simulink model "Lab1"  (R2021a)
settings: Solver=VariableStepAuto  StartTime=0.0  StopTime=8  RelTol=1e-3
undefined symbols (not defined in the file or in its folder): square
libraries: simulink x4
settings Model: Creator=alsin  LastModifiedBy=yasse

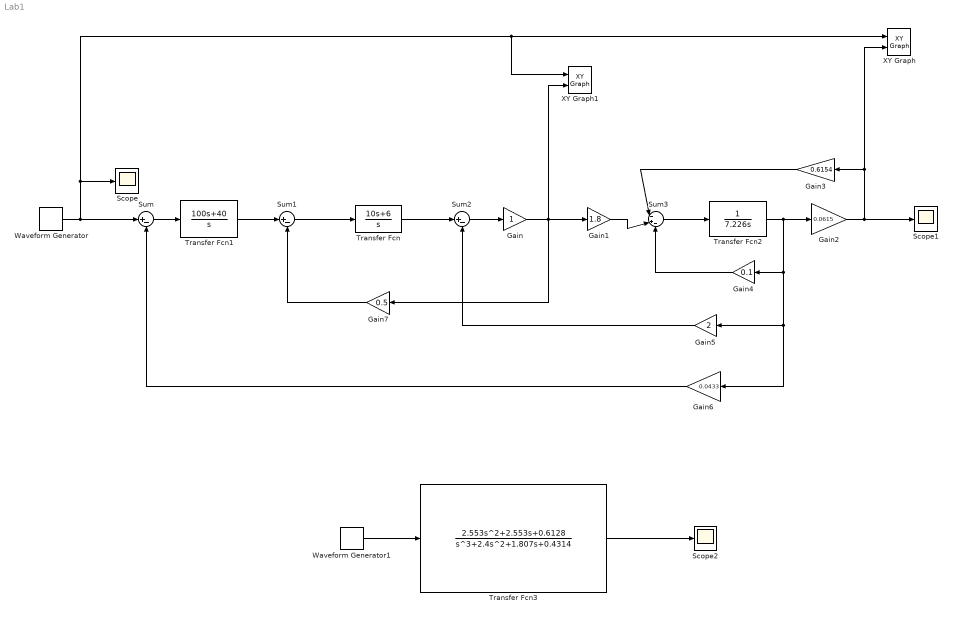
== system Lab1 ==
  Gain : Gain
  Gain1 : Gain  Gain=1.8
  Gain2 : Gain  Gain=0.0615
  Gain3 : Gain  Gain=0.6154
  Gain4 : Gain  Gain=0.1
  Gain5 : Gain  Gain=2
  Gain6 : Gain  Gain=0.0433
  Gain7 : Gain  Gain=0.5
  Scope : Scope
  Scope1 : Scope
  Scope2 : Scope
  Sum : Sum  Inputs=|+-
  Sum1 : Sum  Inputs=|+-
  Sum2 : Sum  Inputs=|+-
  Sum3 : Sum  Inputs=|-+-
  Transfer Fcn : TransferFcn  Numerator=[10 6]  Denominator=[1 0]  ContinuousStateAttributes='KaGtc'
  Transfer Fcn1 : TransferFcn  Numerator=[100 40]  Denominator=[1 0]  ContinuousStateAttributes='Gsc'
  Transfer Fcn2 : TransferFcn  Numerator=[0 1]  Denominator=[7.226 0]
  Transfer Fcn3 : TransferFcn  Numerator=[0 2.553 2.553 0.6128]  Denominator=[1 2.4 1.807 0.4314]
  Waveform Generator : simulink/Sources/Waveform Generator  OutMin=[]  OutMax=[]  OutDataTypeStr=double  SelectedSignal=1  Signals=square(5,31.42,0,80)  BlockNames=MultiportSwitch_ce04f6e477244c1  SampleTime=0.01
  Waveform Generator1 : simulink/Sources/Waveform Generator  OutMin=[]  OutMax=[]  OutDataTypeStr=double  SelectedSignal=1  Signals=sin('Amplitude',4,'Frequency', 200,'Phase', pi/2)  BlockNames=MultiportSwitch_f0c3a2bd8e974ff  SampleTime=0.1
  XY Graph : simulink/Sinks/XY Graph  xmin=-5  xmax=5  ymin=-5  ymax=5  st=0.1
  XY Graph1 : simulink/Sinks/XY Graph  xmin=-5  xmax=5  ymin=-1000  ymax=1000  st=-1
  wires:
  Sum/1 -> Transfer Fcn1/1
  Transfer Fcn1/1 -> Sum1/1
  Sum1/1 -> Transfer Fcn/1
  Transfer Fcn/1 -> Sum2/1
  Sum2/1 -> Gain/1
  Gain1/1 -> Sum3/2
  Sum3/1 -> Transfer Fcn2/1
  Transfer Fcn2/1 -> Gain6/1, Gain5/1, Gain4/1, Gain2/1
  Gain2/1 -> Scope1/1, XY Graph/2, Gain3/1
  Gain3/1 -> Sum3/1
  Gain4/1 -> Sum3/3
  Gain5/1 -> Sum2/2
  Gain6/1 -> Sum/2
  Gain7/1 -> Sum1/2
  Waveform Generator/1 -> XY Graph1/1, XY Graph/1, Scope/1, Sum/1
  Gain/1 -> XY Graph1/2, Gain7/1, Gain1/1
  Transfer Fcn3/1 -> Scope2/1
  Waveform Generator1/1 -> Transfer Fcn3/1
